simulink model "Part2_2"  (R2022a)
settings: Solver=VariableStepAuto  StartTime=0.0  StopTime=1000  RelTol=1e-3
values from neighbouring files (symbols this model uses):
  D = diag([0.01, 0.01, 0.01])    [driver2.m]    (also in driver2_2.m; driver2_3.m; driver_2_2.m)
  g = [0,0,-9.81]    [driver2.m]    (also in driver2_2.m; driver2_3.m; driver_2_2.m)
  I = diag([3e-6, 3e-6, 1e-5])    [driver2.m]    (also in driver2_2.m; driver2_3.m; driver_2_2.m)
  In = inv(I)    [driver2.m]    (also in driver2_2.m; driver2_3.m; driver_2_2.m)
  k = 0.01    [driver2.m]    (also in driver2_2.m; driver2_3.m; driver_2_2.m)
  m = 0.5    [driver2.m]    (also in driver2_2.m; driver2_3.m; driver_2_2.m)
  omg_vec = [0 ... (first row only)    [driver2.m]    (also in driver2_2.m; driver2_3.m; driver_2_2.m)
  tau = [L*k*(Omega(1)^2 - Omega(3)^2) ... (first row only)    [driver2.m]    (also in driver2_2.m; driver2_3.m = 2*w0*[L*k*(Omega(1) - Omega(3)); driver_2_2.m)
libraries: matrix_library x1
settings Model: Creator=askeo  LastModifiedBy=askeo

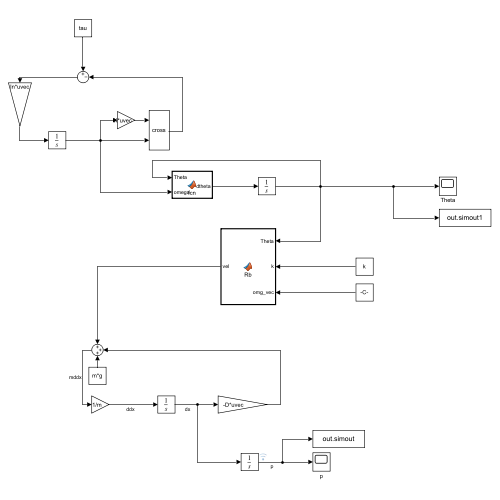
[thumbnail: Simulink's stored preview of the top-level diagram]
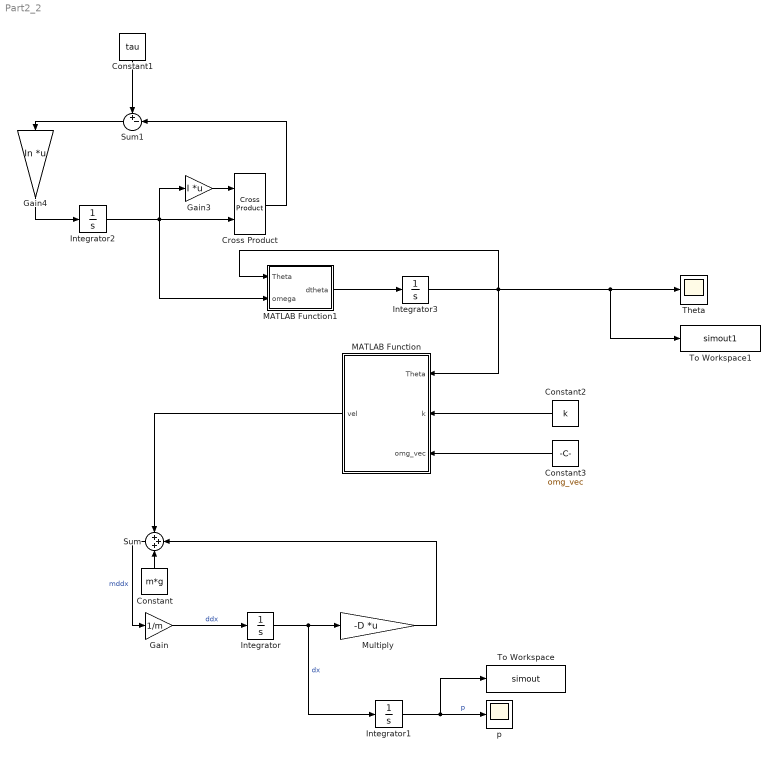
== system Part2_2 ==
  Constant : Constant  Value=m*g
  Constant1 : Constant  Value=tau
  Constant2 : Constant  Value=k
  Constant3 : Constant  Value=omg_vec
  Cross Product : matrix_library/Cross Product
      settings: SourceProductBaseCode=SL
  Gain : Gain  Gain=1/m
  Gain3 : Gain  Gain=I  Multiplication=Matrix(K*u) (u vector)
  Gain4 : Gain  Gain=In  Multiplication=Matrix(K*u) (u vector)
  Integrator : Integrator  InitialCondition=[0;0;0]
  Integrator1 : Integrator  InitialCondition=[0;0;0]
  Integrator2 : Integrator  InitialCondition=[0;0;0]
  Integrator3 : Integrator  InitialCondition=[0; 0; 0]
  MATLAB Function : MATLAB Function  TreatAsAtomicUnit=on
  MATLAB Function1 : MATLAB Function  TreatAsAtomicUnit=on
  Multiply : Gain  Gain=-D  Multiplication=Matrix(K*u) (u vector)
  Sum : Sum  Inputs=+++
  Sum1 : Sum  Inputs=+-|
  Theta : Scope
  To Workspace : ToWorkspace  VariableName=simout  SaveFormat=Timeseries  SampleTime=-1
  To Workspace1 : ToWorkspace  VariableName=simout1  SaveFormat=Timeseries  SampleTime=-1
  p : Scope
  wires:
  Gain/1 -> Integrator/1  "ddx"
  Gain4/1 -> Integrator2/1
  MATLAB Function1/1(dtheta) -> Integrator3/1
  Gain3/1 -> Cross Product/1
  Sum/1 -> Gain/1  "mddx"
  Sum1/1 -> Gain4/1
  Constant1/1 -> Sum1/1
  Multiply/1 -> Sum/2
  Cross Product/1 -> Sum1/2
  Constant/1 -> Sum/3
  Integrator3/1 -> MATLAB Function1/1(Theta), MATLAB Function/1(Theta), To Workspace1/1, Theta/1
  Integrator1/1 -> To Workspace/1, p/1  "p"
  Integrator2/1 -> MATLAB Function1/2(omega), Gain3/1, Cross Product/2
  Integrator/1 -> Integrator1/1, Multiply/1  "dx"
  MATLAB Function/1(vel) -> Sum/1
  Constant2/1 -> MATLAB Function/2(k)
  Constant3/1 -> MATLAB Function/3(omg_vec)

== matlab function Part2_2/MATLAB Function1 ==
  data: dtheta output; Theta input; omega input
function dtheta = fcn(Theta, omega)

C = [1, 0, -sin(Theta(2))
    0, cos(Theta(1)), cos(Theta(2))*sin(Theta(1))
    0, -sin(Theta(1)), cos(Theta(2))*cos(Theta(1))];

dtheta = inv(C)*omega;
end

== matlab function Part2_2/MATLAB Function ==
  data: Theta input; vel output; k input; omg_vec input
function vel = Rb(Theta,k,omg_vec)

q = [(cos(Theta(1)/2) + cos(Theta(2)/2) + cos(Theta(3)/2)), sin(Theta(1)/2), sin(Theta(2)/2), sin(Theta(3)/2)];
q_i = [(cos(Theta(1)/2) + cos(Theta(2)/2) + cos(Theta(3)/2)), -sin(Theta(1)/2), -sin(Theta(2)/2), -sin(Theta(3)/2)]/sum(q.^2);
%q_i = quatinv(q);
q_norm = q/sum(q.^2);
%q_inorm = q_i/sum(q_i.^2);

temp = k*q_i*omg_vec*q_norm';
vel = temp(2:4,1);

end
